simulink model "Planning"  (R2024b)
settings: Solver=FixedStepAuto  StartTime=0.0  StopTime=10.0  RelTol=1e-3
settings Model: DataDictionary=DataDictionary.sldd  Creator=csamak  LastModifiedBy=tsamak
settings OptimizationCC: ZeroExternalMemoryAtStartup=off  ZeroInternalMemoryAtStartup=off  InitFltsAndDblsToZero=on
settings HardwareCC: ProdLongLongMode=on  TargetLongLongMode=on
settings RTWCC: TargetLang=C++  GenerateGPUCode=CUDA
settings GRTTargetCC: TargetLangStandard=C++11 (ISO)  CodeInterfacePackaging=C++ class

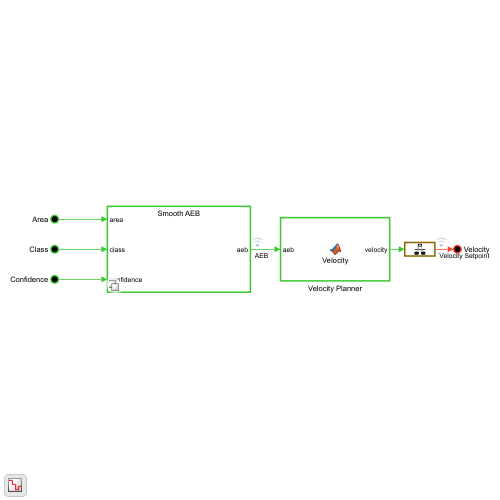
[thumbnail: Simulink's stored preview of the top-level diagram]
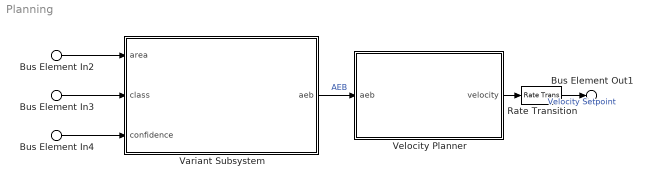
== system Planning ==
  Bus Element In2 : Inport  PortName=Area
  Bus Element In3 : Inport  Port=2  PortName=Class
  Bus Element In4 : Inport  Port=3  PortName=Confidence
  Rate Transition : RateTransition  OutPortSampleTime=0.1
  Variant Subsystem : Subsystem  Variant=on  VariantActivationTime=inherit from Simulink.VariantControl
  Velocity Planner : MATLAB Function  TreatAsAtomicUnit=on
  Bus Element Out1 : Outport  PortName=Velocity
  wires:
  Variant Subsystem/1(aeb) -> Velocity Planner/1(aeb)  "AEB"
  Bus Element In4/1 -> Variant Subsystem/3(confidence)
  Bus Element In3/1 -> Variant Subsystem/2(class)
  Bus Element In2/1 -> Variant Subsystem/1(area)
  Velocity Planner/1(velocity) -> Rate Transition/1
  Rate Transition/1 -> Bus Element Out1/1  "Velocity Setpoint"

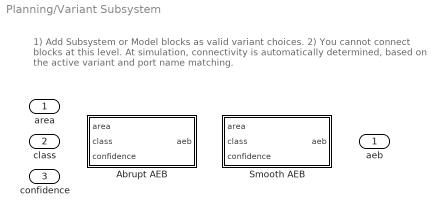
== system Planning/Variant Subsystem ==
  note: 1) Add Subsystem or Model blocks as valid variant choices.
      | 2) You cannot connect blocks at this level. At simulation, connectivity is automatically determined, based on the active variant and port name matching.
  area : Inport
  class : Inport  Port=2
  confidence : Inport  Port=3
  Abrupt AEB : Subsystem  VariantControl=PLANNER==1
  Smooth AEB : Subsystem  VariantControl=PLANNER==2
  aeb : Outport

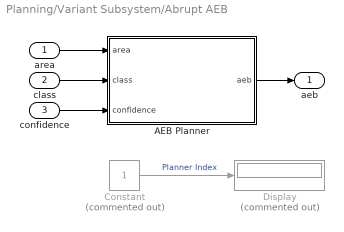
== system Planning/Variant Subsystem/Abrupt AEB ==
  area : Inport
  class : Inport  Port=2
  confidence : Inport  Port=3
  AEB Planner : MATLAB Function  TreatAsAtomicUnit=on
  Constant : Constant  Commented=on
  Display : Display  Commented=on
  aeb : Outport
  wires:
  Constant/1 -> Display/1  "Planner Index"
  confidence/1 -> AEB Planner/3(confidence)
  class/1 -> AEB Planner/2(class)
  area/1 -> AEB Planner/1(area)
  AEB Planner/1(aeb) -> aeb/1

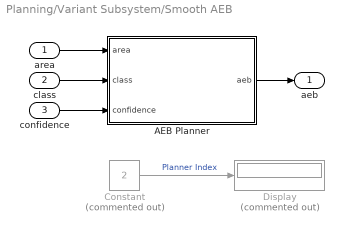
== system Planning/Variant Subsystem/Smooth AEB ==
  area : Inport
  class : Inport  Port=2
  confidence : Inport  Port=3
  AEB Planner : MATLAB Function  TreatAsAtomicUnit=on
  Constant : Constant  Commented=on  Value=2
  Display : Display  Commented=on
  aeb : Outport
  wires:
  Constant/1 -> Display/1  "Planner Index"
  confidence/1 -> AEB Planner/3(confidence)
  class/1 -> AEB Planner/2(class)
  area/1 -> AEB Planner/1(area)
  AEB Planner/1(aeb) -> aeb/1

== matlab function Planning/Variant Subsystem/Smooth AEB/AEB Planner ==
  data: area input; aeb output; class input; confidence input
function aeb = AEB(area, class, confidence)
    aeb = 0;
    valid_classes = [15,16,17,18,19,20,21,22,23,24];
    for i=1:size(area,1)
        if (any(valid_classes(:) == class(i)))
            if (confidence(i) >= 0.5)
                if (area(i) >= 4000)
                    aeb = 0.000025*area(i);
                    aeb = max(0, min(1, aeb));
                end
            end
        end
    end

== matlab function Planning/Variant Subsystem/Abrupt AEB/AEB Planner ==
  data: area input; aeb output; class input; confidence input
function aeb = AEB(area, class, confidence)
    aeb = 0;
    valid_classes = [15,16,17,18,19,20,21,22,23,24];
    for i=1:size(area,1)
        if (any(valid_classes(:) == class(i)))
            if (confidence(i) >= 0.5)
                if (area(i) >= 4000)
                    aeb = 1;
                end
            end
        end
    end

== matlab function Planning/Velocity Planner ==
  data: aeb input; velocity output
function velocity = Velocity(aeb)
    velocity = 0;
    if (aeb >= 0.9)
        velocity = 0;
    else
        velocity = 0.3*(1/(aeb+0.1));
    end
